simulink model "sysgenQAMExt"  (Simulink 7.7)
settings: Solver=ode45  StartTime=0.0  StopTime=3000  RelTol=1e-3
PreLoadFcn:
  | xlrequire('PreLoadFcn')
values from neighbouring files (symbols this model uses):
  hh = hh1/max(hh1)    [sysgenCostasLoop_PreLoadFcn.m]
  j = find(xLabel==')')    [sdspfscope2_r13.m]
  k = (k-1)*3+2    [sdspfscope2_r13.m]
  mu = xfix({xlSigned, 18, 15, xlRound, xlSaturate}, mu)    [lmsErr.m]
undefined symbols (not defined in the file or in its folder): chan, k_i0, k_p0, xlipgetpartsetting, xlsfunxy
libraries: xbsIndex_r4 x477, simulink x2, dspsigops x2, dspmlti4 x2, commchan3 x1, xbsCopyrightNotice_r4 x1, dspobslib x1
(part 4 of 5)

== system sysgenQAMExt/QAM Receiver/QAM Demodulator/Carrier Recovery/Phase Detector/Cordic ==
  x : Inport
  y : Inport  Port=2
  z : Inport  Port=3
  Cordic Fine Angle PE : Subsystem
  Quadrant  Correct : Subsystem
  Quadrant  Map : Subsystem
  x_n : Outport
  y_n : Outport  Port=2
  z_n : Outport  Port=3
  wires:
  Cordic Fine Angle PE/1(x_n) -> x_n/1
  Cordic Fine Angle PE/2(y_n) -> y_n/1
  Cordic Fine Angle PE/3(z_n) -> Quadrant  Correct/1(z_in)
  y/1 -> Quadrant  Map/2(y)
  x/1 -> Quadrant  Map/1(x)
  Quadrant  Map/2(y_map) -> Cordic Fine Angle PE/2(y_0)
  Quadrant  Map/1(x_map) -> Cordic Fine Angle PE/1(x_0)
  Quadrant  Correct/1(z_out) -> z_n/1
  Quadrant  Map/4(z_mux_sel) -> Quadrant  Correct/3(z_mux_sel)
  Quadrant  Map/3(" PI:2_add:sub") -> Quadrant  Correct/2(pi:2_add:sub)
  z/1 -> Cordic Fine Angle PE/3(z_0)

== system sysgenQAMExt/QAM Receiver/QAM Demodulator/Carrier Recovery/Phase Detector/NegB_Cmplx Mult ==
  a_r : Inport
  a_i : Inport  Port=2
  b_r : Inport  Port=3
  b_i : Inport  Port=4
  AddSub : xbsIndex_r4/AddSub  mode=Addition  use_carryin=off  use_carryout=off  en=off  latency=0  precision=User Defined  arith_type="Signed  (2's comp)"  n_bits=lms_mult_post_add_ni  bin_pt=lms_mult_post_add_nf  quantization=Truncate  overflow=Wrap  dbl_ovrd=off  use_behavioral_HDL=on  hw_selection=Fabric  pipelined=off  use_rpm=on  block_type=addsub
      settings: xl_area=[0, 0, 0, 0, 0, 0, 0]  block_version=VER_STRING_GOES_HERE
  AddSub1 : xbsIndex_r4/AddSub  mode=Subtraction  use_carryin=off  use_carryout=off  en=off  latency=0  precision=User Defined  arith_type="Signed  (2's comp)"  n_bits=lms_mult_post_add_ni  bin_pt=lms_mult_post_add_nf  quantization=Truncate  overflow=Wrap  dbl_ovrd=off  use_behavioral_HDL=on  hw_selection=Fabric  pipelined=off  use_rpm=on  block_type=addsub
      settings: xl_area=[0, 0, 0, 0, 0, 0, 0]  block_version=VER_STRING_GOES_HERE
  Mult{1..4} (4 alike) : xbsIndex_r4/Mult  precision=User Defined  arith_type="Signed  (2's comp)"  n_bits=lms_mult_ni  bin_pt=lms_mult_nf  quantization=Truncate  overflow=Wrap  en=off  latency=0  dbl_ovrd=off  use_behavioral_HDL=off  opt=Speed  use_embedded=on  optimum_pipeline=off  pipeline=off  use_rpm=on  placement_style=Rectangular shape  block_type=mult
      settings: infoedit=Multiplies two values.<P><P>Hardware notes: To use the internal pipeline stage of the dedicated multiplier you must select 'Pipeline to Greatest Extent Possible'.  xl_area=[0, 0, 0, 0, 0, 0, 0]  block_version=VER_STRING_GOES_HERE
  p_r : Outport
  p_i : Outport  Port=2
  wires:
  Mult4/1 -> AddSub/1
  a_i/1 -> Mult1/1, Mult3/2
  b_r/1 -> Mult4/2, Mult3/1
  b_i/1 -> Mult1/2, Mult2/2
  a_r/1 -> Mult4/1, Mult2/1
  Mult1/1 -> AddSub/2
  Mult2/1 -> AddSub1/1
  Mult3/1 -> AddSub1/2
  AddSub/1 -> p_r/1
  AddSub1/1 -> p_i/1

== system sysgenQAMExt/QAM Receiver/QAM Demodulator/Carrier Recovery/Phase Detector/Slicer ==
  I_in : Inport
  Q_in : Inport  Port=2
  I Map : Subsystem
  Q Map : Subsystem
  det_ I : Outport
  qntzd_I : Outport  Port=2
  det_Q : Outport  Port=3
  qntzd_Q : Outport  Port=4
  wires:
  Q Map/1(det) -> det_Q/1
  I Map/1(det) -> det_ I/1
  I_in/1 -> I Map/1(x_n)
  Q_in/1 -> Q Map/1(x_n)
  I Map/2(qntzd) -> qntzd_I/1
  Q Map/2(qntzd) -> qntzd_Q/1

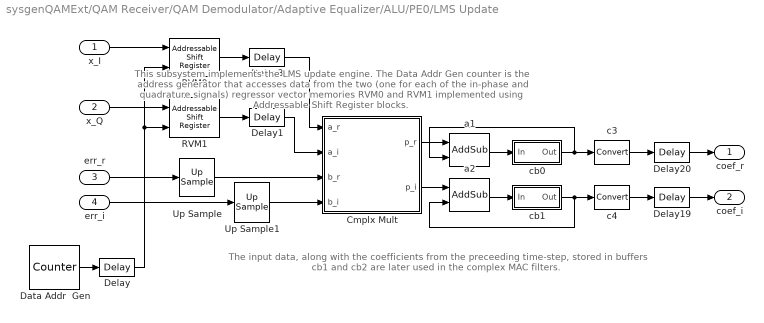
== system sysgenQAMExt/QAM Receiver/QAM Demodulator/Adaptive Equalizer/ALU/PE0/LMS Update ==
  note: This subsystem implements the LMS update engine. The Data Addr Gen
      | counter is the address generator that accesses data from the two (one for each of the
      | in-phase and quadrature signals) regressor vector memories RVM0 and RVM1
      | implemented using Addressable Shift Register blocks.
  note: The input data, along with the coefficients from the
      | preceeding time-step, stored in buffers cb1 and cb2
      | are later used in the complex MAC filters.
  x_I : Inport
  x_Q : Inport  Port=2
  err_r : Inport  Port=3
  err_i : Inport  Port=4
  Cmplx Mult : Subsystem
  Data Addr  Gen : xbsIndex_r4/Counter  cnt_type=Count Limited  cnt_to=3  operation=Up  start_count=0  cnt_by_val=1  arith_type=Unsigned  n_bits=2  bin_pt=0  load_pin=off  rst=off  en=off  explicit_period=off  period=T  dbl_ovrd=off  use_behavioral_HDL=off  implementation=Fabric  use_rpm=off  block_type=counter
      settings: infoedit="Configurable up, down and up/down counter.<P><P>Hardware notes: Free running counters are the least expensive in hardware.  A count limited counter is implemented by combining a counter with a comparator."  xl_area=[0, 0, 0, 0, 0, 0, 0]  block_version=VER_STRING_GOES_HERE
  Delay : xbsIndex_r4/Delay  rst=off  infoeditControl=Selection of Reset will increase slice count due to use of real FFs and instead of SRLs  en=off  latency=1  dbl_ovrd=off  reg_retiming=off  block_type=delay
      settings: infoedit="Delay line having  configurable length.<P><P>Hardware notes: A delay line is a chain, each link of which is an SRL16 followed by a flip-flop. If register retiming is enabled, the delay line is a chain of flip-flops."  xl_area=[0, 0, 0, 0, 0, 0, 0]  block_version=VER_STRING_GOES_HERE
  Delay1 : xbsIndex_r4/Delay  rst=off  infoeditControl=Selection of Reset will increase slice count due to use of real FFs and instead of SRLs  en=off  latency=3  dbl_ovrd=off  reg_retiming=off  block_type=delay
      settings: infoedit="Delay line having  configurable length.<P><P>Hardware notes: A delay line is a chain, each link of which is an SRL16 followed by a flip-flop. If register retiming is enabled, the delay line is a chain of flip-flops."  xl_area=[0, 0, 0, 0, 0, 0, 0]  block_version=VER_STRING_GOES_HERE
  Delay19 : xbsIndex_r4/Delay  rst=off  infoeditControl=Selection of Reset will increase slice count due to use of real FFs and instead of SRLs  en=off  latency=6  dbl_ovrd=off  reg_retiming=off  block_type=delay
      settings: infoedit="Delay line having  configurable length.<P><P>Hardware notes: A delay line is a chain, each link of which is an SRL16 followed by a flip-flop. If register retiming is enabled, the delay line is a chain of flip-flops."  xl_area=[0, 0, 0, 0, 0, 0, 0]  block_version=VER_STRING_GOES_HERE
  Delay20 : xbsIndex_r4/Delay  rst=off  infoeditControl=Selection of Reset will increase slice count due to use of real FFs and instead of SRLs  en=off  latency=6  dbl_ovrd=off  reg_retiming=off  block_type=delay
      settings: infoedit="Delay line having  configurable length.<P><P>Hardware notes: A delay line is a chain, each link of which is an SRL16 followed by a flip-flop. If register retiming is enabled, the delay line is a chain of flip-flops."  xl_area=[0, 0, 0, 0, 0, 0, 0]  block_version=VER_STRING_GOES_HERE
  Delay3 : xbsIndex_r4/Delay  rst=off  infoeditControl=Selection of Reset will increase slice count due to use of real FFs and instead of SRLs  en=off  latency=3  dbl_ovrd=off  reg_retiming=off  block_type=delay
      settings: infoedit="Delay line having  configurable length.<P><P>Hardware notes: A delay line is a chain, each link of which is an SRL16 followed by a flip-flop. If register retiming is enabled, the delay line is a chain of flip-flops."  xl_area=[0, 0, 0, 0, 0, 0, 0]  block_version=VER_STRING_GOES_HERE
  RVM0 : xbsIndex_r4/Addressable Shift Register  infer_latency=off  depth=4  initVector=[0]  en=off  dbl_ovrd=off  use_behavioral_HDL=off  Optimization=Resource  use_rpm=off  block_type=addrsr
      settings: infoedit="Delay of configurable length.  Any element in the delay line can be addressed and driven onto the output port.<P><P>Hardware notes: Implemented using SRL16s.  If a Virtex-II device is used, multiple SRLC16s are cascaded together."  xl_area=[0, 0, 0, 0, 0, 0, 0]  block_version=VER_STRING_GOES_HERE
  RVM1 : xbsIndex_r4/Addressable Shift Register  infer_latency=off  depth=4  initVector=[0]  en=off  dbl_ovrd=off  use_behavioral_HDL=off  Optimization=Resource  use_rpm=off  block_type=addrsr
      settings: infoedit="Delay of configurable length.  Any element in the delay line can be addressed and driven onto the output port.<P><P>Hardware notes: Implemented using SRL16s.  If a Virtex-II device is used, multiple SRLC16s are cascaded together."  xl_area=[0, 0, 0, 0, 0, 0, 0]  block_version=VER_STRING_GOES_HERE
  Up Sample : xbsIndex_r4/Up Sample  sample_ratio=4  copy_samples=on  en=off  latency=0  dbl_ovrd=off  block_type=usamp
      settings: infoedit="Up samples input data.  Inserted values  can be zeros or copies of the most recent input sample.<P><P>Hardware notes: No hardware is needed if inserted values are copies of the input sample; otherwise, a mux and single bit flip-flop are used."  xl_area=[0, 0, 0, 0, 0, 0, 0]  block_version=VER_STRING_GOES_HERE
  Up Sample1 : xbsIndex_r4/Up Sample  sample_ratio=4  copy_samples=on  en=off  latency=0  dbl_ovrd=off  block_type=usamp
      settings: infoedit="Up samples input data.  Inserted values  can be zeros or copies of the most recent input sample.<P><P>Hardware notes: No hardware is needed if inserted values are copies of the input sample; otherwise, a mux and single bit flip-flop are used."  xl_area=[0, 0, 0, 0, 0, 0, 0]  block_version=VER_STRING_GOES_HERE
  a1 : xbsIndex_r4/AddSub  mode=Addition  use_carryin=off  use_carryout=off  en=off  latency=0  precision=User Defined  arith_type="Signed  (2's comp)"  n_bits=lms_acc_ni  bin_pt=lms_acc_nf  quantization="Round  (unbiased: +/- Inf)"  overflow=Wrap  dbl_ovrd=off  use_behavioral_HDL=on  hw_selection=Fabric  pipelined=off  use_rpm=on  block_type=addsub
      settings: xl_area=[0, 0, 0, 0, 0, 0, 0]  block_version=VER_STRING_GOES_HERE
  a2 : xbsIndex_r4/AddSub  mode=Addition  use_carryin=off  use_carryout=off  en=off  latency=0  precision=User Defined  arith_type="Signed  (2's comp)"  n_bits=lms_acc_ni  bin_pt=lms_acc_nf  quantization="Round  (unbiased: +/- Inf)"  overflow=Wrap  dbl_ovrd=off  use_behavioral_HDL=on  hw_selection=Fabric  pipelined=off  use_rpm=on  block_type=addsub
      settings: xl_area=[0, 0, 0, 0, 0, 0, 0]  block_version=VER_STRING_GOES_HERE
  c3 : xbsIndex_r4/Convert  gui_display_data_type=Fixed-point  arith_type="Signed  (2's comp)"  n_bits=coeff_ni  bin_pt=coeff_nf  float_type=Single  exp_bits=8  fraction_bits=24  quantization="Round  (unbiased: +/- Inf)"  overflow=Wrap  en=off  latency=0  dbl_ovrd=off  pipeline=off  block_type=convert
      settings: infoedit=The input is presented at the output after quantization and overflow effects.<P><P>Hardware notes: Additional hardware is used when rounding or saturation is selected and output width is less than the input width.  xl_area=[0, 0, 0, 0, 0, 0, 0]  block_version=VER_STRING_GOES_HERE
  c4 : xbsIndex_r4/Convert  gui_display_data_type=Fixed-point  arith_type="Signed  (2's comp)"  n_bits=coeff_ni  bin_pt=coeff_nf  float_type=Single  exp_bits=8  fraction_bits=24  quantization="Round  (unbiased: +/- Inf)"  overflow=Wrap  en=off  latency=0  dbl_ovrd=off  pipeline=off  block_type=convert
      settings: infoedit=The input is presented at the output after quantization and overflow effects.<P><P>Hardware notes: Additional hardware is used when rounding or saturation is selected and output width is less than the input width.  xl_area=[0, 0, 0, 0, 0, 0, 0]  block_version=VER_STRING_GOES_HERE
  cb0 : Subsystem
  cb1 : Subsystem
  coef_r : Outport
  coef_i : Outport  Port=2
  wires:
  x_I/1 -> RVM0/1
  RVM0/1 -> Delay3/1
  x_Q/1 -> RVM1/1
  RVM1/1 -> Delay1/1
  Delay3/1 -> Cmplx Mult/1(a_r)
  Delay1/1 -> Cmplx Mult/2(a_i)
  a1/1 -> cb0/1(In)
  a2/1 -> cb1/1(In)
  cb0/1(Out) -> c3/1, a1/2
  cb1/1(Out) -> c4/1, a2/2
  err_r/1 -> Up Sample/1
  err_i/1 -> Up Sample1/1
  Up Sample/1 -> Cmplx Mult/3(b_r)
  Up Sample1/1 -> Cmplx Mult/4(b_i)
  Data Addr  Gen/1 -> Delay/1
  Delay/1 -> RVM1/2, RVM0/2
  c3/1 -> Delay20/1
  c4/1 -> Delay19/1
  Delay19/1 -> coef_i/1
  Delay20/1 -> coef_r/1
  Cmplx Mult/1(p_r) -> a1/1
  Cmplx Mult/2(p_i) -> a2/1

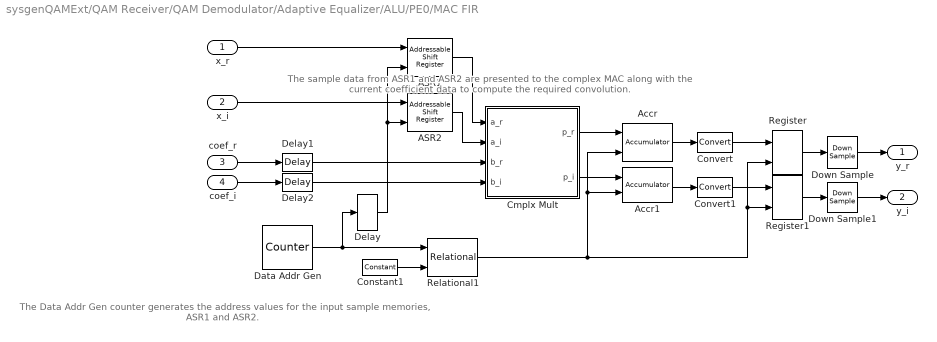
== system sysgenQAMExt/QAM Receiver/QAM Demodulator/Adaptive Equalizer/ALU/PE0/MAC FIR ==
  note: The sample data from ASR1 and ASR2 are presented to the
      | complex MAC along with the current coefficient  data to compute
      | the required convolution.
  note: The Data Addr Gen counter generates the address values for
      | the input sample memories, ASR1 and ASR2.
  x_r : Inport
  x_i : Inport  Port=2
  coef_r : Inport  Port=3
  coef_i : Inport  Port=4
  ASR1 : xbsIndex_r4/Addressable Shift Register  infer_latency=off  depth=4  initVector=[0]  en=off  dbl_ovrd=off  use_behavioral_HDL=off  Optimization=Resource  use_rpm=off  block_type=addrsr
      settings: infoedit="Delay of configurable length.  Any element in the delay line can be addressed and driven onto the output port.<P><P>Hardware notes: Implemented using SRL16s.  If a Virtex-II device is used, multiple SRLC16s are cascaded together."  xl_area=[0, 0, 0, 0, 0, 0, 0]  block_version=VER_STRING_GOES_HERE
  ASR2 : xbsIndex_r4/Addressable Shift Register  infer_latency=off  depth=4  initVector=[0]  en=off  dbl_ovrd=off  use_behavioral_HDL=off  Optimization=Resource  use_rpm=off  block_type=addrsr
      settings: infoedit="Delay of configurable length.  Any element in the delay line can be addressed and driven onto the output port.<P><P>Hardware notes: Implemented using SRL16s.  If a Virtex-II device is used, multiple SRLC16s are cascaded together."  xl_area=[0, 0, 0, 0, 0, 0, 0]  block_version=VER_STRING_GOES_HERE
  Accr : xbsIndex_r4/Accumulator  operation=Add  n_bits=46  overflow=Wrap  scale=1  rst=on  hasbypass=on  en=off  dbl_ovrd=off  use_behavioral_HDL=on  implementation=Fabric  block_type=accum
      settings: infoedit="Adder or subtractor-based accumulator.   Output type and binary point position match the input.<P><P>Hardware notes: When \"Reinitialize with Input 'b' on Reset\" is selected, the accumulator is forced to run at the system rate even if the input 'b' is running at a slower rate."  xl_area=[0, 0, 0, 0, 0, 0, 0]  block_version=VER_STRING_GOES_HERE
  Accr1 : xbsIndex_r4/Accumulator  operation=Add  n_bits=46  overflow=Wrap  scale=1  rst=on  hasbypass=on  en=off  dbl_ovrd=off  use_behavioral_HDL=on  implementation=Fabric  block_type=accum
      settings: infoedit="Adder or subtractor-based accumulator.   Output type and binary point position match the input.<P><P>Hardware notes: When \"Reinitialize with Input 'b' on Reset\" is selected, the accumulator is forced to run at the system rate even if the input 'b' is running at a slower rate."  xl_area=[0, 0, 0, 0, 0, 0, 0]  block_version=VER_STRING_GOES_HERE
  Cmplx Mult : Subsystem
  Constant1 : xbsIndex_r4/Constant  const=0  gui_display_data_type=Fixed-point  arith_type=Unsigned  n_bits=1  bin_pt=0  preci_type=Single  exp_width=8  frac_width=24  explicit_period=on  period=T  equ=P=C  opselect=C  inp2=PCIN>>17  opr=+  inp1=P  carry=CIN  dbl_ovrd=off  block_type=constant
      settings: block_version=VER_STRING_GOES_HERE
  Convert : xbsIndex_r4/Convert  gui_display_data_type=Fixed-point  arith_type="Signed  (2's comp)"  n_bits=24  bin_pt=20  float_type=Single  exp_bits=8  fraction_bits=24  quantization="Round  (unbiased: +/- Inf)"  overflow=Wrap  en=off  latency=0  dbl_ovrd=off  pipeline=off  block_type=convert
      settings: infoedit=The input is presented at the output after quantization and overflow effects.<P><P>Hardware notes: Additional hardware is used when rounding or saturation is selected and output width is less than the input width.  xl_area=[0, 0, 0, 0, 0, 0, 0]  block_version=VER_STRING_GOES_HERE
  Convert1 : xbsIndex_r4/Convert  gui_display_data_type=Fixed-point  arith_type="Signed  (2's comp)"  n_bits=24  bin_pt=20  float_type=Single  exp_bits=8  fraction_bits=24  quantization="Round  (unbiased: +/- Inf)"  overflow=Wrap  en=off  latency=0  dbl_ovrd=off  pipeline=off  block_type=convert
      settings: infoedit=The input is presented at the output after quantization and overflow effects.<P><P>Hardware notes: Additional hardware is used when rounding or saturation is selected and output width is less than the input width.  xl_area=[0, 0, 0, 0, 0, 0, 0]  block_version=VER_STRING_GOES_HERE
  Data Addr Gen : xbsIndex_r4/Counter  cnt_type=Count Limited  cnt_to=3  operation=Up  start_count=0  cnt_by_val=1  arith_type=Unsigned  n_bits=2  bin_pt=0  load_pin=off  rst=off  en=off  explicit_period=off  period=T  dbl_ovrd=off  use_behavioral_HDL=off  implementation=Fabric  use_rpm=off  block_type=counter
      settings: infoedit="Configurable up, down and up/down counter.<P><P>Hardware notes: Free running counters are the least expensive in hardware.  A count limited counter is implemented by combining a counter with a comparator."  xl_area=[0, 0, 0, 0, 0, 0, 0]  block_version=VER_STRING_GOES_HERE
  Delay : xbsIndex_r4/Delay  rst=off  infoeditControl=Selection of Reset will increase slice count due to use of real FFs and instead of SRLs  en=off  latency=1  dbl_ovrd=off  reg_retiming=off  block_type=delay
      settings: infoedit="Delay line having  configurable length.<P><P>Hardware notes: A delay line is a chain, each link of which is an SRL16 followed by a flip-flop. If register retiming is enabled, the delay line is a chain of flip-flops."  xl_area=[0, 0, 0, 0, 0, 0, 0]  block_version=VER_STRING_GOES_HERE
  Delay1 : xbsIndex_r4/Delay  rst=off  infoeditControl=Selection of Reset will increase slice count due to use of real FFs and instead of SRLs  en=off  latency=1  dbl_ovrd=off  reg_retiming=off  block_type=delay
      settings: infoedit="Delay line having  configurable length.<P><P>Hardware notes: A delay line is a chain, each link of which is an SRL16 followed by a flip-flop. If register retiming is enabled, the delay line is a chain of flip-flops."  xl_area=[0, 0, 0, 0, 0, 0, 0]  block_version=VER_STRING_GOES_HERE
  Delay2 : xbsIndex_r4/Delay  rst=off  infoeditControl=Selection of Reset will increase slice count due to use of real FFs and instead of SRLs  en=off  latency=1  dbl_ovrd=off  reg_retiming=off  block_type=delay
      settings: infoedit="Delay line having  configurable length.<P><P>Hardware notes: A delay line is a chain, each link of which is an SRL16 followed by a flip-flop. If register retiming is enabled, the delay line is a chain of flip-flops."  xl_area=[0, 0, 0, 0, 0, 0, 0]  block_version=VER_STRING_GOES_HERE
  Down Sample : xbsIndex_r4/Down Sample  sample_ratio=4  sample_phase="Last Value of Frame  (most efficient)"  en=off  latency=1  dbl_ovrd=off  block_type=dsamp
      settings: xl_area=[0, 0, 0, 0, 0, 0, 0]  block_version=VER_STRING_GOES_HERE
  Down Sample1 : xbsIndex_r4/Down Sample  sample_ratio=4  sample_phase="Last Value of Frame  (most efficient)"  en=off  latency=1  dbl_ovrd=off  block_type=dsamp
      settings: xl_area=[0, 0, 0, 0, 0, 0, 0]  block_version=VER_STRING_GOES_HERE
  Register : xbsIndex_r4/Register  init=0  rst=off  en=on  dbl_ovrd=off  block_type=register
      settings: xl_area=[0, 0, 0, 0, 0, 0, 0]  block_version=VER_STRING_GOES_HERE
  Register1 : xbsIndex_r4/Register  init=0  rst=off  en=on  dbl_ovrd=off  block_type=register
      settings: xl_area=[0, 0, 0, 0, 0, 0, 0]  block_version=VER_STRING_GOES_HERE
  Relational1 : xbsIndex_r4/Relational  mode=a=b  en=off  latency=7  dbl_ovrd=off  block_type=relational
      settings: xl_area=[0, 0, 0, 0, 0, 0, 0]  block_version=VER_STRING_GOES_HERE
  y_r : Outport
  y_i : Outport  Port=2
  wires:
  Delay/1 -> ASR1/2, ASR2/2
  x_r/1 -> ASR1/1
  ASR1/1 -> Cmplx Mult/1(a_r)
  x_i/1 -> ASR2/1
  ASR2/1 -> Cmplx Mult/2(a_i)
  coef_r/1 -> Delay1/1
  coef_i/1 -> Delay2/1
  Delay2/1 -> Cmplx Mult/4(b_i)
  Delay1/1 -> Cmplx Mult/3(b_r)
  Accr/1 -> Convert/1
  Cmplx Mult/1(p_r) -> Accr/1
  Cmplx Mult/2(p_i) -> Accr1/1
  Accr1/1 -> Convert1/1
  Relational1/1 -> Accr/2, Accr1/2, Register/2, Register1/2
  Register/1 -> Down Sample/1
  Register1/1 -> Down Sample1/1
  Convert/1 -> Register/1
  Convert1/1 -> Register1/1
  Down Sample/1 -> y_r/1
  Down Sample1/1 -> y_i/1
  Data Addr Gen/1 -> Relational1/1, Delay/1
  Constant1/1 -> Relational1/2

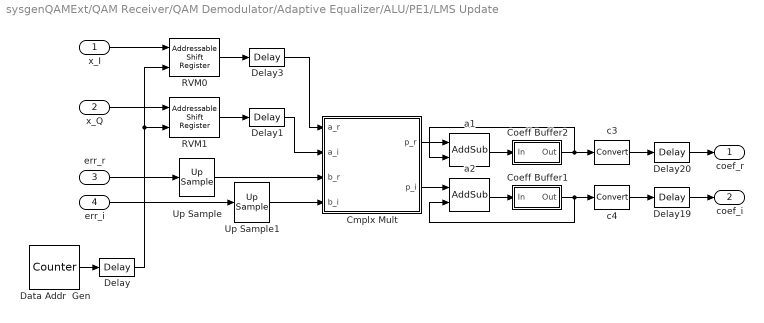
== system sysgenQAMExt/QAM Receiver/QAM Demodulator/Adaptive Equalizer/ALU/PE1/LMS Update ==
  x_I : Inport
  x_Q : Inport  Port=2
  err_r : Inport  Port=3
  err_i : Inport  Port=4
  Cmplx Mult : Subsystem
  Coeff Buffer1 : Subsystem
  Coeff Buffer2 : Subsystem
  Data Addr  Gen : xbsIndex_r4/Counter  cnt_type=Count Limited  cnt_to=3  operation=Up  start_count=0  cnt_by_val=1  arith_type=Unsigned  n_bits=2  bin_pt=0  load_pin=off  rst=off  en=off  explicit_period=off  period=T  dbl_ovrd=off  use_behavioral_HDL=off  implementation=Fabric  use_rpm=off  block_type=counter
      settings: infoedit="Configurable up, down and up/down counter.<P><P>Hardware notes: Free running counters are the least expensive in hardware.  A count limited counter is implemented by combining a counter with a comparator."  xl_area=[0, 0, 0, 0, 0, 0, 0]  block_version=VER_STRING_GOES_HERE
  Delay : xbsIndex_r4/Delay  rst=off  infoeditControl=Selection of Reset will increase slice count due to use of real FFs and instead of SRLs  en=off  latency=1  dbl_ovrd=off  reg_retiming=off  block_type=delay
      settings: infoedit="Delay line having  configurable length.<P><P>Hardware notes: A delay line is a chain, each link of which is an SRL16 followed by a flip-flop. If register retiming is enabled, the delay line is a chain of flip-flops."  xl_area=[0, 0, 0, 0, 0, 0, 0]  block_version=VER_STRING_GOES_HERE
  Delay1 : xbsIndex_r4/Delay  rst=off  infoeditControl=Selection of Reset will increase slice count due to use of real FFs and instead of SRLs  en=off  latency=3  dbl_ovrd=off  reg_retiming=off  block_type=delay
      settings: infoedit="Delay line having  configurable length.<P><P>Hardware notes: A delay line is a chain, each link of which is an SRL16 followed by a flip-flop. If register retiming is enabled, the delay line is a chain of flip-flops."  xl_area=[0, 0, 0, 0, 0, 0, 0]  block_version=VER_STRING_GOES_HERE
  Delay19 : xbsIndex_r4/Delay  rst=off  infoeditControl=Selection of Reset will increase slice count due to use of real FFs and instead of SRLs  en=off  latency=6  dbl_ovrd=off  reg_retiming=off  block_type=delay
      settings: infoedit="Delay line having  configurable length.<P><P>Hardware notes: A delay line is a chain, each link of which is an SRL16 followed by a flip-flop. If register retiming is enabled, the delay line is a chain of flip-flops."  xl_area=[0, 0, 0, 0, 0, 0, 0]  block_version=VER_STRING_GOES_HERE
  Delay20 : xbsIndex_r4/Delay  rst=off  infoeditControl=Selection of Reset will increase slice count due to use of real FFs and instead of SRLs  en=off  latency=6  dbl_ovrd=off  reg_retiming=off  block_type=delay
      settings: infoedit="Delay line having  configurable length.<P><P>Hardware notes: A delay line is a chain, each link of which is an SRL16 followed by a flip-flop. If register retiming is enabled, the delay line is a chain of flip-flops."  xl_area=[0, 0, 0, 0, 0, 0, 0]  block_version=VER_STRING_GOES_HERE
  Delay3 : xbsIndex_r4/Delay  rst=off  infoeditControl=Selection of Reset will increase slice count due to use of real FFs and instead of SRLs  en=off  latency=3  dbl_ovrd=off  reg_retiming=off  block_type=delay
      settings: infoedit="Delay line having  configurable length.<P><P>Hardware notes: A delay line is a chain, each link of which is an SRL16 followed by a flip-flop. If register retiming is enabled, the delay line is a chain of flip-flops."  xl_area=[0, 0, 0, 0, 0, 0, 0]  block_version=VER_STRING_GOES_HERE
  RVM0 : xbsIndex_r4/Addressable Shift Register  infer_latency=off  depth=4  initVector=[0]  en=off  dbl_ovrd=off  use_behavioral_HDL=off  Optimization=Resource  use_rpm=off  block_type=addrsr
      settings: infoedit="Delay of configurable length.  Any element in the delay line can be addressed and driven onto the output port.<P><P>Hardware notes: Implemented using SRL16s.  If a Virtex-II device is used, multiple SRLC16s are cascaded together."  xl_area=[0, 0, 0, 0, 0, 0, 0]  block_version=VER_STRING_GOES_HERE
  RVM1 : xbsIndex_r4/Addressable Shift Register  infer_latency=off  depth=4  initVector=[0]  en=off  dbl_ovrd=off  use_behavioral_HDL=off  Optimization=Resource  use_rpm=off  block_type=addrsr
      settings: infoedit="Delay of configurable length.  Any element in the delay line can be addressed and driven onto the output port.<P><P>Hardware notes: Implemented using SRL16s.  If a Virtex-II device is used, multiple SRLC16s are cascaded together."  xl_area=[0, 0, 0, 0, 0, 0, 0]  block_version=VER_STRING_GOES_HERE
  Up Sample : xbsIndex_r4/Up Sample  sample_ratio=4  copy_samples=on  en=off  latency=0  dbl_ovrd=off  block_type=usamp
      settings: infoedit="Up samples input data.  Inserted values  can be zeros or copies of the most recent input sample.<P><P>Hardware notes: No hardware is needed if inserted values are copies of the input sample; otherwise, a mux and single bit flip-flop are used."  xl_area=[0, 0, 0, 0, 0, 0, 0]  block_version=VER_STRING_GOES_HERE
  Up Sample1 : xbsIndex_r4/Up Sample  sample_ratio=4  copy_samples=on  en=off  latency=0  dbl_ovrd=off  block_type=usamp
      settings: infoedit="Up samples input data.  Inserted values  can be zeros or copies of the most recent input sample.<P><P>Hardware notes: No hardware is needed if inserted values are copies of the input sample; otherwise, a mux and single bit flip-flop are used."  xl_area=[0, 0, 0, 0, 0, 0, 0]  block_version=VER_STRING_GOES_HERE
  a1 : xbsIndex_r4/AddSub  mode=Addition  use_carryin=off  use_carryout=off  en=off  latency=0  precision=User Defined  arith_type="Signed  (2's comp)"  n_bits=lms_acc_ni  bin_pt=lms_acc_nf  quantization="Round  (unbiased: +/- Inf)"  overflow=Wrap  dbl_ovrd=off  use_behavioral_HDL=on  hw_selection=Fabric  pipelined=off  use_rpm=on  block_type=addsub
      settings: xl_area=[0, 0, 0, 0, 0, 0, 0]  block_version=VER_STRING_GOES_HERE
  a2 : xbsIndex_r4/AddSub  mode=Addition  use_carryin=off  use_carryout=off  en=off  latency=0  precision=User Defined  arith_type="Signed  (2's comp)"  n_bits=lms_acc_ni  bin_pt=lms_acc_nf  quantization="Round  (unbiased: +/- Inf)"  overflow=Wrap  dbl_ovrd=off  use_behavioral_HDL=on  hw_selection=Fabric  pipelined=off  use_rpm=on  block_type=addsub
      settings: xl_area=[0, 0, 0, 0, 0, 0, 0]  block_version=VER_STRING_GOES_HERE
  c3 : xbsIndex_r4/Convert  gui_display_data_type=Fixed-point  arith_type="Signed  (2's comp)"  n_bits=coeff_ni  bin_pt=coeff_nf  float_type=Single  exp_bits=8  fraction_bits=24  quantization="Round  (unbiased: +/- Inf)"  overflow=Wrap  en=off  latency=0  dbl_ovrd=off  pipeline=off  block_type=convert
      settings: infoedit=The input is presented at the output after quantization and overflow effects.<P><P>Hardware notes: Additional hardware is used when rounding or saturation is selected and output width is less than the input width.  xl_area=[0, 0, 0, 0, 0, 0, 0]  block_version=VER_STRING_GOES_HERE
  c4 : xbsIndex_r4/Convert  gui_display_data_type=Fixed-point  arith_type="Signed  (2's comp)"  n_bits=coeff_ni  bin_pt=coeff_nf  float_type=Single  exp_bits=8  fraction_bits=24  quantization="Round  (unbiased: +/- Inf)"  overflow=Wrap  en=off  latency=0  dbl_ovrd=off  pipeline=off  block_type=convert
      settings: infoedit=The input is presented at the output after quantization and overflow effects.<P><P>Hardware notes: Additional hardware is used when rounding or saturation is selected and output width is less than the input width.  xl_area=[0, 0, 0, 0, 0, 0, 0]  block_version=VER_STRING_GOES_HERE
  coef_r : Outport
  coef_i : Outport  Port=2
  wires:
  x_I/1 -> RVM0/1
  RVM0/1 -> Delay3/1
  x_Q/1 -> RVM1/1
  RVM1/1 -> Delay1/1
  Delay3/1 -> Cmplx Mult/1(a_r)
  Delay1/1 -> Cmplx Mult/2(a_i)
  a1/1 -> Coeff Buffer2/1(In)
  a2/1 -> Coeff Buffer1/1(In)
  Coeff Buffer2/1(Out) -> c3/1, a1/2
  Coeff Buffer1/1(Out) -> c4/1, a2/2
  err_r/1 -> Up Sample/1
  err_i/1 -> Up Sample1/1
  Up Sample/1 -> Cmplx Mult/3(b_r)
  Up Sample1/1 -> Cmplx Mult/4(b_i)
  Data Addr  Gen/1 -> Delay/1
  Delay/1 -> RVM1/2, RVM0/2
  c3/1 -> Delay20/1
  c4/1 -> Delay19/1
  Delay19/1 -> coef_i/1
  Delay20/1 -> coef_r/1
  Cmplx Mult/1(p_r) -> a1/1
  Cmplx Mult/2(p_i) -> a2/1

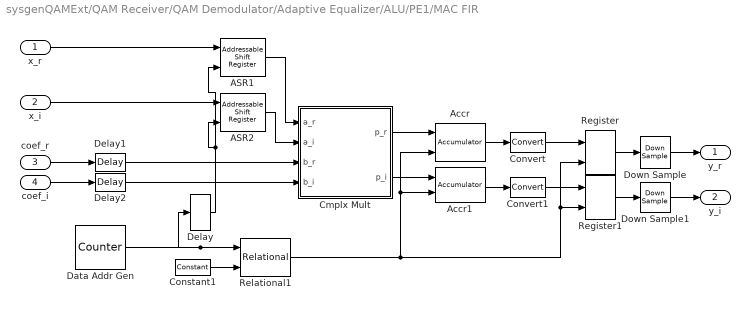
== system sysgenQAMExt/QAM Receiver/QAM Demodulator/Adaptive Equalizer/ALU/PE1/MAC FIR ==
  x_r : Inport
  x_i : Inport  Port=2
  coef_r : Inport  Port=3
  coef_i : Inport  Port=4
  ASR1 : xbsIndex_r4/Addressable Shift Register  infer_latency=off  depth=4  initVector=[0]  en=off  dbl_ovrd=off  use_behavioral_HDL=off  Optimization=Resource  use_rpm=off  block_type=addrsr
      settings: infoedit="Delay of configurable length.  Any element in the delay line can be addressed and driven onto the output port.<P><P>Hardware notes: Implemented using SRL16s.  If a Virtex-II device is used, multiple SRLC16s are cascaded together."  xl_area=[0, 0, 0, 0, 0, 0, 0]  block_version=VER_STRING_GOES_HERE
  ASR2 : xbsIndex_r4/Addressable Shift Register  infer_latency=off  depth=4  initVector=[0]  en=off  dbl_ovrd=off  use_behavioral_HDL=off  Optimization=Resource  use_rpm=off  block_type=addrsr
      settings: infoedit="Delay of configurable length.  Any element in the delay line can be addressed and driven onto the output port.<P><P>Hardware notes: Implemented using SRL16s.  If a Virtex-II device is used, multiple SRLC16s are cascaded together."  xl_area=[0, 0, 0, 0, 0, 0, 0]  block_version=VER_STRING_GOES_HERE
  Accr : xbsIndex_r4/Accumulator  operation=Add  n_bits=46  overflow=Wrap  scale=1  rst=on  hasbypass=on  en=off  dbl_ovrd=off  use_behavioral_HDL=on  implementation=Fabric  block_type=accum
      settings: infoedit="Adder or subtractor-based accumulator.   Output type and binary point position match the input.<P><P>Hardware notes: When \"Reinitialize with Input 'b' on Reset\" is selected, the accumulator is forced to run at the system rate even if the input 'b' is running at a slower rate."  xl_area=[0, 0, 0, 0, 0, 0, 0]  block_version=VER_STRING_GOES_HERE
  Accr1 : xbsIndex_r4/Accumulator  operation=Add  n_bits=46  overflow=Wrap  scale=1  rst=on  hasbypass=on  en=off  dbl_ovrd=off  use_behavioral_HDL=on  implementation=Fabric  block_type=accum
      settings: infoedit="Adder or subtractor-based accumulator.   Output type and binary point position match the input.<P><P>Hardware notes: When \"Reinitialize with Input 'b' on Reset\" is selected, the accumulator is forced to run at the system rate even if the input 'b' is running at a slower rate."  xl_area=[0, 0, 0, 0, 0, 0, 0]  block_version=VER_STRING_GOES_HERE
  Cmplx Mult : Subsystem
  Constant1 : xbsIndex_r4/Constant  const=0  gui_display_data_type=Fixed-point  arith_type=Unsigned  n_bits=1  bin_pt=0  preci_type=Single  exp_width=8  frac_width=24  explicit_period=on  period=T  equ=P=C  opselect=C  inp2=PCIN>>17  opr=+  inp1=P  carry=CIN  dbl_ovrd=off  block_type=constant
      settings: block_version=VER_STRING_GOES_HERE
  Convert : xbsIndex_r4/Convert  gui_display_data_type=Fixed-point  arith_type="Signed  (2's comp)"  n_bits=24  bin_pt=20  float_type=Single  exp_bits=8  fraction_bits=24  quantization="Round  (unbiased: +/- Inf)"  overflow=Wrap  en=off  latency=0  dbl_ovrd=off  pipeline=off  block_type=convert
      settings: infoedit=The input is presented at the output after quantization and overflow effects.<P><P>Hardware notes: Additional hardware is used when rounding or saturation is selected and output width is less than the input width.  xl_area=[0, 0, 0, 0, 0, 0, 0]  block_version=VER_STRING_GOES_HERE
  Convert1 : xbsIndex_r4/Convert  gui_display_data_type=Fixed-point  arith_type="Signed  (2's comp)"  n_bits=24  bin_pt=20  float_type=Single  exp_bits=8  fraction_bits=24  quantization="Round  (unbiased: +/- Inf)"  overflow=Wrap  en=off  latency=0  dbl_ovrd=off  pipeline=off  block_type=convert
      settings: infoedit=The input is presented at the output after quantization and overflow effects.<P><P>Hardware notes: Additional hardware is used when rounding or saturation is selected and output width is less than the input width.  xl_area=[0, 0, 0, 0, 0, 0, 0]  block_version=VER_STRING_GOES_HERE
  Data Addr Gen : xbsIndex_r4/Counter  cnt_type=Count Limited  cnt_to=3  operation=Up  start_count=0  cnt_by_val=1  arith_type=Unsigned  n_bits=2  bin_pt=0  load_pin=off  rst=off  en=off  explicit_period=off  period=T  dbl_ovrd=off  use_behavioral_HDL=off  implementation=Fabric  use_rpm=off  block_type=counter
      settings: infoedit="Configurable up, down and up/down counter.<P><P>Hardware notes: Free running counters are the least expensive in hardware.  A count limited counter is implemented by combining a counter with a comparator."  xl_area=[0, 0, 0, 0, 0, 0, 0]  block_version=VER_STRING_GOES_HERE
  Delay : xbsIndex_r4/Delay  rst=off  infoeditControl=Selection of Reset will increase slice count due to use of real FFs and instead of SRLs  en=off  latency=1  dbl_ovrd=off  reg_retiming=off  block_type=delay
      settings: infoedit="Delay line having  configurable length.<P><P>Hardware notes: A delay line is a chain, each link of which is an SRL16 followed by a flip-flop. If register retiming is enabled, the delay line is a chain of flip-flops."  xl_area=[0, 0, 0, 0, 0, 0, 0]  block_version=VER_STRING_GOES_HERE
  Delay1 : xbsIndex_r4/Delay  rst=off  infoeditControl=Selection of Reset will increase slice count due to use of real FFs and instead of SRLs  en=off  latency=1  dbl_ovrd=off  reg_retiming=off  block_type=delay
      settings: infoedit="Delay line having  configurable length.<P><P>Hardware notes: A delay line is a chain, each link of which is an SRL16 followed by a flip-flop. If register retiming is enabled, the delay line is a chain of flip-flops."  xl_area=[0, 0, 0, 0, 0, 0, 0]  block_version=VER_STRING_GOES_HERE
  Delay2 : xbsIndex_r4/Delay  rst=off  infoeditControl=Selection of Reset will increase slice count due to use of real FFs and instead of SRLs  en=off  latency=1  dbl_ovrd=off  reg_retiming=off  block_type=delay
      settings: infoedit="Delay line having  configurable length.<P><P>Hardware notes: A delay line is a chain, each link of which is an SRL16 followed by a flip-flop. If register retiming is enabled, the delay line is a chain of flip-flops."  xl_area=[0, 0, 0, 0, 0, 0, 0]  block_version=VER_STRING_GOES_HERE
  Down Sample : xbsIndex_r4/Down Sample  sample_ratio=4  sample_phase="Last Value of Frame  (most efficient)"  en=off  latency=1  dbl_ovrd=off  block_type=dsamp
      settings: xl_area=[0, 0, 0, 0, 0, 0, 0]  block_version=VER_STRING_GOES_HERE
  Down Sample1 : xbsIndex_r4/Down Sample  sample_ratio=4  sample_phase="Last Value of Frame  (most efficient)"  en=off  latency=1  dbl_ovrd=off  block_type=dsamp
      settings: xl_area=[0, 0, 0, 0, 0, 0, 0]  block_version=VER_STRING_GOES_HERE
  Register : xbsIndex_r4/Register  init=0  rst=off  en=on  dbl_ovrd=off  block_type=register
      settings: xl_area=[0, 0, 0, 0, 0, 0, 0]  block_version=VER_STRING_GOES_HERE
  Register1 : xbsIndex_r4/Register  init=0  rst=off  en=on  dbl_ovrd=off  block_type=register
      settings: xl_area=[0, 0, 0, 0, 0, 0, 0]  block_version=VER_STRING_GOES_HERE
  Relational1 : xbsIndex_r4/Relational  mode=a=b  en=off  latency=7  dbl_ovrd=off  block_type=relational
      settings: xl_area=[0, 0, 0, 0, 0, 0, 0]  block_version=VER_STRING_GOES_HERE
  y_r : Outport
  y_i : Outport  Port=2
  wires:
  Delay/1 -> ASR1/2, ASR2/2
  x_r/1 -> ASR1/1
  ASR1/1 -> Cmplx Mult/1(a_r)
  x_i/1 -> ASR2/1
  ASR2/1 -> Cmplx Mult/2(a_i)
  coef_r/1 -> Delay1/1
  coef_i/1 -> Delay2/1
  Delay2/1 -> Cmplx Mult/4(b_i)
  Delay1/1 -> Cmplx Mult/3(b_r)
  Accr/1 -> Convert/1
  Cmplx Mult/1(p_r) -> Accr/1
  Cmplx Mult/2(p_i) -> Accr1/1
  Accr1/1 -> Convert1/1
  Relational1/1 -> Accr/2, Accr1/2, Register/2, Register1/2
  Register/1 -> Down Sample/1
  Register1/1 -> Down Sample1/1
  Convert/1 -> Register/1
  Convert1/1 -> Register1/1
  Down Sample/1 -> y_r/1
  Down Sample1/1 -> y_i/1
  Data Addr Gen/1 -> Relational1/1, Delay/1
  Constant1/1 -> Relational1/2

== system sysgenQAMExt/QAM Receiver/QAM Demodulator/Carrier Recovery/Phase Detector/Cordic/Cordic Fine Angle PE ==
  note: The CORDIC processor uses a fully unfolded architecture, using 5 iterations
      | and 11-bit precision input samples.  Bit-growth to the final output precision of
      | 16-bits is permitted.
  x_0 : Inport
  y_0 : Inport  Port=2
  z_0 : Inport  Port=3
  Cordic PE0 : Subsystem
  Cordic PE1 : Subsystem
  Cordic PE2 : Subsystem
  Cordic PE3 : Subsystem
  Cordic PE4 : Subsystem
  x_n : Outport
  y_n : Outport  Port=2
  z_n : Outport  Port=3
  wires:
  Cordic PE4/3(z) -> z_n/1
  Cordic PE4/2(y) -> y_n/1
  Cordic PE4/1(x) -> x_n/1
  Cordic PE2/3(z) -> Cordic PE3/3(z_n-1)
  Cordic PE2/2(y) -> Cordic PE3/2(y_n-1)
  Cordic PE2/1(x) -> Cordic PE3/1(x_n-1)
  Cordic PE1/3(z) -> Cordic PE2/3(z_n-1)
  Cordic PE1/2(y) -> Cordic PE2/2(y_n-1)
  Cordic PE1/1(x) -> Cordic PE2/1(x_n-1)
  Cordic PE0/3(z) -> Cordic PE1/3(z_n-1)
  Cordic PE0/2(y) -> Cordic PE1/2(y_n-1)
  Cordic PE0/1(x) -> Cordic PE1/1(x_n-1)
  z_0/1 -> Cordic PE0/3(z_n-1)
  y_0/1 -> Cordic PE0/2(y_n-1)
  x_0/1 -> Cordic PE0/1(x_n-1)
  Cordic PE3/1(x) -> Cordic PE4/1(x_n-1)
  Cordic PE3/2(y) -> Cordic PE4/2(y_n-1)
  Cordic PE3/3(z) -> Cordic PE4/3(z_n-1)

== system sysgenQAMExt/QAM Receiver/QAM Demodulator/Carrier Recovery/Phase Detector/Cordic/Quadrant  Correct ==
  z_in : Inport
  pi:2_add:sub : Inport  Port=2
  z_mux_sel : Inport  Port=3
  AddSub1 : xbsIndex_r4/AddSub  mode=Addition or Subtraction  use_carryin=off  use_carryout=off  en=off  latency=0  precision=User Defined  arith_type="Signed  (2's comp)"  n_bits=atan_nbits  bin_pt=atan_nbits_frac  quantization=Truncate  overflow=Wrap  dbl_ovrd=off  use_behavioral_HDL=on  hw_selection=Fabric  pipelined=off  use_rpm=off  block_type=addsub
      settings: xl_area=[0, 0, 0, 0, 0, 0, 0]  block_version=VER_STRING_GOES_HERE
  Mux : xbsIndex_r4/Mux  inputs=2  en=off  latency=0  precision=Full  arith_type="Signed  (2's comp)"  n_bits=8  bin_pt=2  quantization=Truncate  overflow=Wrap  dbl_ovrd=off  block_type=mux
      settings: xl_area=[0, 0, 0, 0, 0, 0, 0]  block_version=VER_STRING_GOES_HERE
  PI:2 : xbsIndex_r4/Constant  const=pi/2  gui_display_data_type=Fixed-point  arith_type=Signed (2's comp)  n_bits=atan_nbits  bin_pt=atan_nbits_frac  preci_type=Single  exp_width=8  frac_width=24  explicit_period=off  period=1  equ=P=C  opselect=C  inp2=PCIN>>17  opr=+  inp1=P  carry=CIN  dbl_ovrd=off  block_type=constant
      settings: block_version=VER_STRING_GOES_HERE
  z_out : Outport
  wires:
  z_mux_sel/1 -> Mux/1
  AddSub1/1 -> Mux/3
  PI:2/1 -> AddSub1/2
  pi:2_add:sub/1 -> AddSub1/3
  Mux/1 -> z_out/1
  z_in/1 -> AddSub1/1, Mux/2

== system sysgenQAMExt/QAM Receiver/QAM Demodulator/Carrier Recovery/Phase Detector/Cordic/Quadrant  Map ==
  x : Inport
  y : Inport  Port=2
  Concat : xbsIndex_r4/Concat  num_inputs=2  dbl_ovrd=off  block_type=concat
      settings: block_version=VER_STRING_GOES_HERE
  Mux : xbsIndex_r4/Mux  inputs=3  en=off  latency=0  precision=User Defined  arith_type="Signed  (2's comp)"  n_bits=cordic_pe_nbits_total  bin_pt=cordic_pe_nbits_frac  quantization=Truncate  overflow=Wrap  dbl_ovrd=off  block_type=mux
      settings: xl_area=[0, 0, 0, 0, 0, 0, 0]  block_version=VER_STRING_GOES_HERE
  Mux1 : xbsIndex_r4/Mux  inputs=3  en=off  latency=0  precision=User Defined  arith_type="Signed  (2's comp)"  n_bits=cordic_pe_nbits_total  bin_pt=cordic_pe_nbits_frac  quantization=Truncate  overflow=Wrap  dbl_ovrd=off  block_type=mux
      settings: xl_area=[0, 0, 0, 0, 0, 0, 0]  block_version=VER_STRING_GOES_HERE
  Negate : xbsIndex_r4/Negate  precision=User Defined  arith_type=Unsigned  n_bits=cordic_pe_nbits_total  bin_pt=cordic_pe_nbits_frac  quantization=Truncate  overflow=Wrap  en=off  latency=0  dbl_ovrd=off  block_type=negate
      settings: xl_area=[0, 0, 0, 0, 0, 0, 0]  block_version=VER_STRING_GOES_HERE
  Negate1 : xbsIndex_r4/Negate  precision=User Defined  arith_type=Unsigned  n_bits=cordic_pe_nbits_total  bin_pt=cordic_pe_nbits_frac  quantization=Truncate  overflow=Wrap  en=off  latency=0  dbl_ovrd=off  block_type=negate
      settings: xl_area=[0, 0, 0, 0, 0, 0, 0]  block_version=VER_STRING_GOES_HERE
  ROM : xbsIndex_r4/ROM  depth=4  initVector=[0 1 0 2]  distributed_mem=Distributed memory  rst=off  init_reg=0  en=off  latency=0  gui_display_data_type=Fixed-point  arith_type=Unsigned  n_bits=2  bin_pt=0  preci_type=Single  exp_width=8  frac_width=24  dbl_ovrd=off  optimize=Area  use_rpm=off  block_type=sprom
      settings: xl_area=[0, 0, 0, 0, 0, 0, 0]  block_version=VER_STRING_GOES_HERE
  sgn(x) : xbsIndex_r4/Slice  nbits=1  boolean_output=on  mode=Upper Bit Location + Width  bit1=0  base1=MSB of Input  bit0=0  base0=LSB of Input  dbl_ovrd=off  block_type=slice
      settings: infoedit="Extracts a given range of bits from each input sample and presents it at the output.  The output type is ordinarily unsigned with binary point at zero, but can be Boolean when the slice is one bit wide.<P><P>Hardware notes: In hardware this block costs nothing."  block_version=VER_STRING_GOES_HERE
  sgn(y) : xbsIndex_r4/Slice  nbits=1  boolean_output=on  mode=Upper Bit Location + Width  bit1=0  base1=MSB of Input  bit0=0  base0=LSB of Input  dbl_ovrd=off  block_type=slice
      settings: infoedit="Extracts a given range of bits from each input sample and presents it at the output.  The output type is ordinarily unsigned with binary point at zero, but can be Boolean when the slice is one bit wide.<P><P>Hardware notes: In hardware this block costs nothing."  block_version=VER_STRING_GOES_HERE
  x_map : Outport
  y_map : Outport  Port=2
  " PI:2_add:sub" : Outport  Port=3
  z_mux_sel : Outport  Port=4
  wires:
  ROM/1 -> Mux1/1, Mux/1
  Concat/1 -> ROM/1
  sgn(x)/1 -> z_mux_sel/1, Concat/2
  sgn(y)/1 -> " PI:2_add:sub"/1, Concat/1
  Negate1/1 -> Mux/4
  Negate/1 -> Mux1/3
  Mux1/1 -> y_map/1
  Mux/1 -> x_map/1
  y/1 -> Negate1/1, Mux/3, Mux1/2, sgn(y)/1
  x/1 -> Negate/1, Mux1/4, sgn(x)/1, Mux/2

== system sysgenQAMExt/QAM Receiver/QAM Demodulator/Carrier Recovery/Phase Detector/Slicer/I Map ==
  x_n : Inport
  Concat : xbsIndex_r4/Concat  num_inputs=2  dbl_ovrd=off  block_type=concat
      settings: block_version=VER_STRING_GOES_HERE
  Mux : xbsIndex_r4/Mux  inputs=2  en=off  latency=0  precision=Full  arith_type="Signed  (2's comp)"  n_bits=8  bin_pt=2  quantization=Truncate  overflow=Wrap  dbl_ovrd=off  block_type=mux
      settings: xl_area=[0, 0, 0, 0, 0, 0, 0]  block_version=VER_STRING_GOES_HERE
  Negate : xbsIndex_r4/Negate  precision=Full  arith_type=Unsigned  n_bits=16  bin_pt=12  quantization=Truncate  overflow=Wrap  en=off  latency=0  dbl_ovrd=off  block_type=negate
      settings: xl_area=[0, 0, 0, 0, 0, 0, 0]  block_version=VER_STRING_GOES_HERE
  ROM : xbsIndex_r4/ROM  depth=4  initVector=[1/3 1 -1/3 -1]  distributed_mem=Distributed memory  rst=off  init_reg=0  en=off  latency=0  gui_display_data_type=Fixed-point  arith_type="Signed  (2's comp)"  n_bits=16  bin_pt=15  preci_type=Single  exp_width=8  frac_width=24  dbl_ovrd=off  optimize=Area  use_rpm=on  block_type=sprom
      settings: xl_area=[0, 0, 0, 0, 0, 0, 0]  block_version=VER_STRING_GOES_HERE
  ROM1 : xbsIndex_r4/ROM  depth=4  initVector=[.5 1 -.5 -1]  distributed_mem=Distributed memory  rst=off  init_reg=0  en=off  latency=0  gui_display_data_type=Fixed-point  arith_type="Signed  (2's comp)"  n_bits=3  bin_pt=1  preci_type=Single  exp_width=8  frac_width=24  dbl_ovrd=off  optimize=Area  use_rpm=on  block_type=sprom
      settings: xl_area=[0, 0, 0, 0, 0, 0, 0]  block_version=VER_STRING_GOES_HERE
  Relational : xbsIndex_r4/Relational  mode=a<b  en=off  latency=0  dbl_ovrd=off  block_type=relational
      settings: xl_area=[0, 0, 0, 0, 0, 0, 0]  block_version=VER_STRING_GOES_HERE
  Relational1 : xbsIndex_r4/Relational  mode=a>=b  en=off  latency=0  dbl_ovrd=off  block_type=relational
      settings: xl_area=[0, 0, 0, 0, 0, 0, 0]  block_version=VER_STRING_GOES_HERE
  Slice : xbsIndex_r4/Slice  nbits=1  boolean_output=off  mode=Upper Bit Location + Width  bit1=0  base1=MSB of Input  bit0=0  base0=LSB of Input  dbl_ovrd=off  block_type=slice
      settings: infoedit="Extracts a given range of bits from each input sample and presents it at the output.  The output type is ordinarily unsigned with binary point at zero, but can be Boolean when the slice is one bit wide.<P><P>Hardware notes: In hardware this block costs nothing."  block_version=VER_STRING_GOES_HERE
  k1 : xbsIndex_r4/Constant  const=2/3  gui_display_data_type=Fixed-point  arith_type=Unsigned  n_bits=8  bin_pt=8  preci_type=Single  exp_width=8  frac_width=24  explicit_period=off  period=1  equ=P=C  opselect=C  inp2=PCIN>>17  opr=+  inp1=P  carry=CIN  dbl_ovrd=off  block_type=constant
      settings: block_version=VER_STRING_GOES_HERE
  k2 : xbsIndex_r4/Constant  const=0  gui_display_data_type=Fixed-point  arith_type=Unsigned  n_bits=8  bin_pt=0  preci_type=Single  exp_width=8  frac_width=24  explicit_period=off  period=1  equ=P=C  opselect=C  inp2=PCIN>>17  opr=+  inp1=P  carry=CIN  dbl_ovrd=off  block_type=constant
      settings: block_version=VER_STRING_GOES_HERE
  det : Outport
  qntzd : Outport  Port=2
  wires:
  Slice/1 -> Mux/1
  x_n/1 -> Slice/1, Negate/1, Mux/2, Relational1/2
  Negate/1 -> Mux/3
  Mux/1 -> Relational/2
  k2/1 -> Relational1/1
  Relational/1 -> Concat/2
  Relational1/1 -> Concat/1
  Concat/1 -> ROM/1, ROM1/1
  ROM/1 -> det/1
  k1/1 -> Relational/1
  ROM1/1 -> qntzd/1

== system sysgenQAMExt/QAM Receiver/QAM Demodulator/Carrier Recovery/Phase Detector/Slicer/Q Map ==
  x_n : Inport
  Concat : xbsIndex_r4/Concat  num_inputs=2  dbl_ovrd=off  block_type=concat
      settings: block_version=VER_STRING_GOES_HERE
  Mux : xbsIndex_r4/Mux  inputs=2  en=off  latency=0  precision=Full  arith_type="Signed  (2's comp)"  n_bits=8  bin_pt=2  quantization=Truncate  overflow=Wrap  dbl_ovrd=off  block_type=mux
      settings: xl_area=[0, 0, 0, 0, 0, 0, 0]  block_version=VER_STRING_GOES_HERE
  Negate : xbsIndex_r4/Negate  precision=Full  arith_type=Unsigned  n_bits=16  bin_pt=12  quantization=Truncate  overflow=Wrap  en=off  latency=0  dbl_ovrd=off  block_type=negate
      settings: xl_area=[0, 0, 0, 0, 0, 0, 0]  block_version=VER_STRING_GOES_HERE
  ROM : xbsIndex_r4/ROM  depth=4  initVector=[1/3 1 -1/3 -1]  distributed_mem=Distributed memory  rst=off  init_reg=0  en=off  latency=0  gui_display_data_type=Fixed-point  arith_type="Signed  (2's comp)"  n_bits=16  bin_pt=15  preci_type=Single  exp_width=8  frac_width=24  dbl_ovrd=off  optimize=Area  use_rpm=on  block_type=sprom
      settings: xl_area=[0, 0, 0, 0, 0, 0, 0]  block_version=VER_STRING_GOES_HERE
  ROM1 : xbsIndex_r4/ROM  depth=4  initVector=[.5 1 -.5 -1]  distributed_mem=Distributed memory  rst=off  init_reg=0  en=off  latency=0  gui_display_data_type=Fixed-point  arith_type="Signed  (2's comp)"  n_bits=3  bin_pt=1  preci_type=Single  exp_width=8  frac_width=24  dbl_ovrd=off  optimize=Area  use_rpm=on  block_type=sprom
      settings: xl_area=[0, 0, 0, 0, 0, 0, 0]  block_version=VER_STRING_GOES_HERE
  Relational : xbsIndex_r4/Relational  mode=a<b  en=off  latency=0  dbl_ovrd=off  block_type=relational
      settings: xl_area=[0, 0, 0, 0, 0, 0, 0]  block_version=VER_STRING_GOES_HERE
  Relational1 : xbsIndex_r4/Relational  mode=a>=b  en=off  latency=0  dbl_ovrd=off  block_type=relational
      settings: xl_area=[0, 0, 0, 0, 0, 0, 0]  block_version=VER_STRING_GOES_HERE
  Slice : xbsIndex_r4/Slice  nbits=1  boolean_output=off  mode=Upper Bit Location + Width  bit1=0  base1=MSB of Input  bit0=0  base0=LSB of Input  dbl_ovrd=off  block_type=slice
      settings: infoedit="Extracts a given range of bits from each input sample and presents it at the output.  The output type is ordinarily unsigned with binary point at zero, but can be Boolean when the slice is one bit wide.<P><P>Hardware notes: In hardware this block costs nothing."  block_version=VER_STRING_GOES_HERE
  k1 : xbsIndex_r4/Constant  const=2/3  gui_display_data_type=Fixed-point  arith_type=Unsigned  n_bits=8  bin_pt=8  preci_type=Single  exp_width=8  frac_width=24  explicit_period=off  period=1  equ=P=C  opselect=C  inp2=PCIN>>17  opr=+  inp1=P  carry=CIN  dbl_ovrd=off  block_type=constant
      settings: block_version=VER_STRING_GOES_HERE
  k2 : xbsIndex_r4/Constant  const=0  gui_display_data_type=Fixed-point  arith_type=Unsigned  n_bits=8  bin_pt=0  preci_type=Single  exp_width=8  frac_width=24  explicit_period=off  period=1  equ=P=C  opselect=C  inp2=PCIN>>17  opr=+  inp1=P  carry=CIN  dbl_ovrd=off  block_type=constant
      settings: block_version=VER_STRING_GOES_HERE
  det : Outport
  qntzd : Outport  Port=2
  wires:
  k1/1 -> Relational/1
  ROM/1 -> det/1
  Concat/1 -> ROM/1, ROM1/1
  Relational1/1 -> Concat/1
  Relational/1 -> Concat/2
  k2/1 -> Relational1/1
  Mux/1 -> Relational/2
  Negate/1 -> Mux/3
  x_n/1 -> Relational1/2, Mux/2, Negate/1, Slice/1
  Slice/1 -> Mux/1
  ROM1/1 -> qntzd/1
